simulink library "fastled"  (R2020b)
settings: Solver=VariableStepAuto  StartTime=0.0  StopTime=10.0  RelTol=1e-3
settings Model: Creator=brianhannan  LastModifiedBy=brianhannan

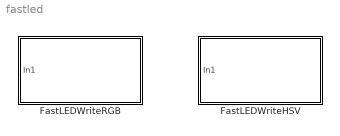
== system fastled ==
  FastLEDWriteHSV : Subsystem  mask(FastLEDWrite){pinNum=5, numLEDs=3}
      mask prompts: pinNum "Data pin:"; numLEDs "Num. LEDs:"
      mask help: Control a WS2812B LED strip using FastLED and an Arduino Uno.
      mask init:
      | % add 1 to to pinNum b/c starts at 2
      | pinNum = uint8(pinNum + 1);
      | numLEDs = uint8(numLEDs);
      mask TypeOptions pinNum: 2 | 3 | 4 | 5 | 6 | 7 | 8 | 9 | 10 | 11 | 12 | 13
      mask Display: disp('Fast LED Write HSV')
  FastLEDWriteRGB : Subsystem  mask(FastLEDWrite){pinNum=5, numLEDs=3}
      mask prompts: pinNum "Data pin:"; numLEDs "Num. LEDs:"
      mask help: Control a WS2812B LED strip using FastLED and an Arduino Uno.
      mask init:
      | % add 1 to to pinNum b/c starts at 2
      | pinNum = uint8(pinNum + 1);
      | numLEDs = uint8(numLEDs);
      mask TypeOptions pinNum: 2 | 3 | 4 | 5 | 6 | 7 | 8 | 9 | 10 | 11 | 12 | 13
      mask Display: disp('Fast LED Write RGB')

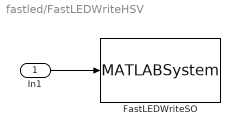
== system fastled/FastLEDWriteHSV ==
  In1 : Inport
  FastLEDWriteSO : MATLABSystem  System=fledblk.FastLEDWriteHSV  Pin=pinNum  NumLEDs=numLEDs
      mask Type: fledblk.FastLEDWriteHSV
      mask Display:
      | disp('FastLED Write');
      | port_label('input',1,'u');
  wires:
  In1/1 -> FastLEDWriteSO/1

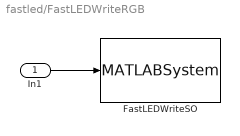
== system fastled/FastLEDWriteRGB ==
  In1 : Inport
  FastLEDWriteSO : MATLABSystem  System=fledblk.FastLEDWriteRGB  Pin=pinNum  NumLEDs=numLEDs
      mask Type: fledblk.FastLEDWriteRGB
      mask Display:
      | disp('FastLED Write');
      | port_label('input',1,'u');
  wires:
  In1/1 -> FastLEDWriteSO/1
